simulink library "COR_lib"  (Simulink 7.4)
settings: Solver=FixedStepDiscrete  StartTime=0.0  StopTime=Inf  FixedStep=0.01  RelTol=1e-3
values from neighbouring files (symbols this model uses):
  CORc_fac_CellRDcse_fault = mpt.Parameter    [COR_CAL.m]
  CORc_fac_CellRDcse_warn = mpt.Parameter    [COR_CAL.m]
  CORc_i_ChaEndCur = mpt.Parameter    [COR_CAL.m]
  CORc_i_SOCCrectCurThrld = mpt.Parameter    [COR_CAL.m]
  CORc_pct_DeltSoe_max = mpt.Parameter    [COR_CAL.m]
  CORc_pct_DeltSoe_min = mpt.Parameter    [COR_CAL.m]
  CORc_pct_SOCModValue = mpt.Parameter    [COR_CAL.m]
  CORc_v_CellVoltMax = mpt.Parameter    [COR_CAL.m]
undefined symbols (not defined in the file or in its folder): BATd_iflt_CellCDcse_fault, BATd_pct_CellCVariMax, BATd_pct_CellCVariMin, BATd_v_CellUpperVolt, BATd_v_PackVoltMin, BATm_c_CellChaC_AH, BATm_c_CellDchC_AH, BATm_e_CellSoe, BATm_e_ChaCellSoe, BATm_e_DchCellSoe, BATm_i_PerChaCur, BATm_i_PerDchCur, BATm_i_PulChaCur_limit, BATm_i_PulDchCur_limit, BATm_i_PulDchVolt_limit, BATm_pct_CellCDcseRatio, BATm_pct_CellCycle, BATm_pct_CellSoc, BATm_pct_ChaCellSoc, BATm_pct_DchCellSoc, BATm_pct_SOCofOCVPct, BATm_pct_SohRatio, BATm_r_ChaDcIR, BATm_r_DchDcIR, BATm_v_CellOCV, BATx_pct_CellSocRatio, BATx_pct_PackSoh, BATx_t_CellChaTemp, BATx_t_CellDchTemp, BATx_tm_OfflineTime, BATy_i_CellChaCur, BATy_i_CellDchCur, BATz_v_CellChaVolt, BATz_v_DchCellVolt, BATz_v_DchCellVoltForSoe, BCU_FastCharge_St, BCU_SlowCharge_St, BMS_Const_TickTm_s, BMU_Run_St, FCM_Charging_St, PACK_Const_CellNumOfMdl, PACK_Const_CellNumOfPack, PACK_Const_CycCnt, PACK_Const_MdlNumOfPack, PACK_Const_ParaCellNumOfMdl, PACK_Const_TempSnrNumOfMdl, SCM_Charging_St
libraries: Defined_Functionality x17
(part 1 of 2)
settings Model: Creator=zhaoxiangri  LastModifiedBy=sunsijun

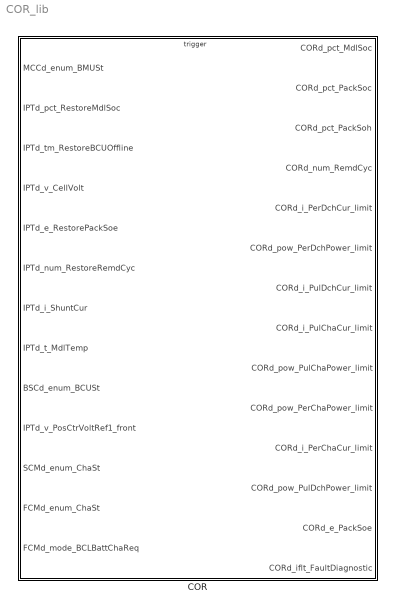
== system COR_lib ==
  COR : Subsystem  TreatAsAtomicUnit=on

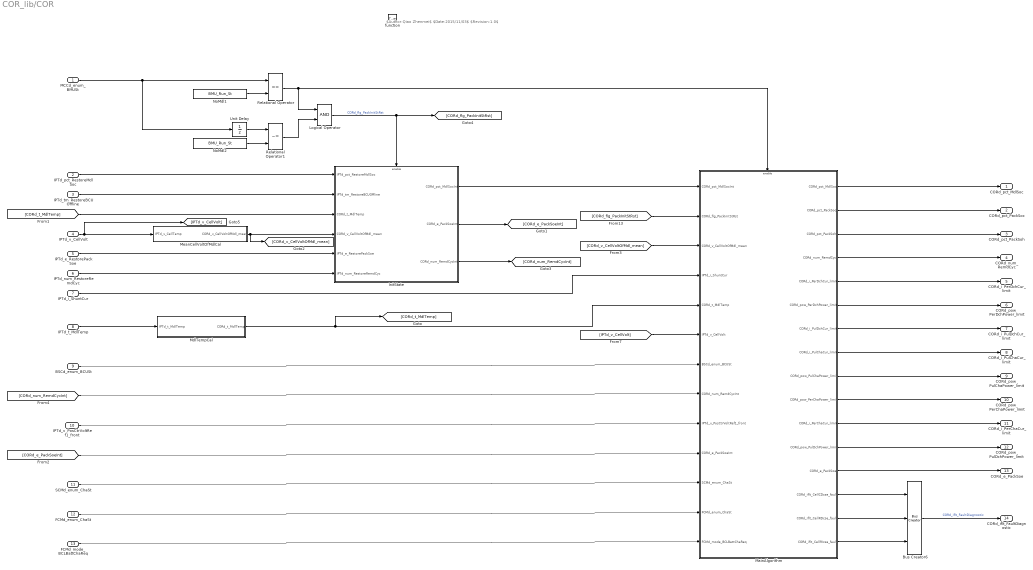
== system COR_lib/COR ==
  note: $Author:Qiao Zhenmei$
      | $Date:2015/11/03$
      | $Revision:1.0$
  MCCd_enum_BMUSt : Inport  OutDataType=sfix(16)  OutScaling=2^0
  IPTd_pct_RestoreMdlSoc : Inport  Port=2  OutDataType=sfix(16)  OutScaling=2^0
  IPTd_tm_RestoreBCUOffline : Inport  Port=3  OutDataType=sfix(16)  OutScaling=2^0
  IPTd_v_CellVolt : Inport  Port=4  OutDataType=sfix(16)  OutScaling=2^0
  IPTd_e_RestorePackSoe : Inport  Port=5  OutDataType=sfix(16)  OutScaling=2^0
  IPTd_num_RestoreRemdCyc : Inport  Port=6  OutDataType=sfix(16)  OutScaling=2^0
  IPTd_i_ShuntCur : Inport  Port=7
  IPTd_t_MdlTemp : Inport  Port=8  DataType=single  OutDataTypeStr=single
  BSCd_enum_BCUSt : Inport  Port=9
  IPTd_v_PosCtrVoltRef1_front : Inport  Port=10  OutDataType=fixdt(1,16,2^-6,0)
  SCMd_enum_ChaSt : Inport  Port=11
  FCMd_enum_ChaSt : Inport  Port=12
  FCMd_mode_BCLBattChaReq : Inport  Port=13
  function : TriggerPort  TriggerType=function-call
  Bus Creator6 : BusCreator  Inputs=3
  InitState : Subsystem
  Logical Operator : Logic  AllPortsSameDT=off  OutDataTypeMode=boolean  LogicDataType=fixdt(0, 8)  OutDataTypeStr=boolean
  MainAlgorithm : Subsystem
  MdlTempCal : Subsystem
  MeanCellVoltOfMdlCal : Subsystem
  NoMdl1 : Constant  Value=BMU_Run_St  OutDataTypeMode=uint8  OutDataType=fixdt(1, 16)  OutScaling=2^0  OutDataTypeStr=uint8
  NoMdl2 : Constant  Value=BMU_Run_St  OutDataTypeMode=uint8  OutDataType=fixdt(1, 16)  OutScaling=2^0  OutDataTypeStr=uint8
  Relational Operator : RelationalOperator  Operator===  LogicOutDataTypeMode=boolean  LogicDataType=fixdt(0, 8)  OutDataTypeStr=boolean
  Relational Operator1 : RelationalOperator  Operator=~=  LogicOutDataTypeMode=boolean  LogicDataType=fixdt(0, 8)  OutDataTypeStr=boolean
  Unit Delay : UnitDelay  SampleTime=-1
  CORd_pct_MdlSoc : Outport  InitialOutput=0
  CORd_pct_PackSoc : Outport  Port=2  InitialOutput=0
  CORd_pct_PackSoh : Outport  Port=3  InitialOutput=0
  CORd_num_RemdCyc : Outport  Port=4
  CORd_i_PerDchCur_limit : Outport  Port=5  InitialOutput=0
  CORd_pow_PerDchPower_limit : Outport  Port=6  InitialOutput=0
  CORd_i_PulDchCur_limit : Outport  Port=7  OutDataType=sfix(16)  OutScaling=2^0  InitialOutput=0
  CORd_i_PulChaCur_limit : Outport  Port=8  OutDataType=sfix(16)  OutScaling=2^0  InitialOutput=0
  CORd_pow_PulChaPower_limit : Outport  Port=9  OutDataType=sfix(16)  OutScaling=2^0  InitialOutput=0
  CORd_pow_PerChaPower_limit : Outport  Port=10  InitialOutput=0
  CORd_i_PerChaCur_limit : Outport  Port=11  InitialOutput=0
  CORd_pow_PulDchPower_limit : Outport  Port=12  OutDataType=sfix(16)  OutScaling=2^0  InitialOutput=0
  CORd_e_PackSoe : Outport  Port=13  InitialOutput=0
  CORd_iflt_FaultDiagnostic : Outport  Port=14
  wires:
  [CORd_num_RemdCycInt] -> MainAlgorithm/8(CORd_num_RemdCycInt)
  InitState/3(CORd_num_RemdCycInt) -> [CORd_num_RemdCycInt]
  [CORd_e_PackSoeInt] -> MainAlgorithm/10(CORd_e_PackSoeInt)
  InitState/2(CORd_e_PackSoeInt) -> [CORd_e_PackSoeInt]
  MainAlgorithm/16(CORd_iflt_CellRIcse_fault) -> Bus Creator6/3
  MainAlgorithm/15(CORd_iflt_CellRDcse_fault) -> Bus Creator6/2
  MainAlgorithm/14(CORd_iflt_CellCDcse_fault) -> Bus Creator6/1
  Relational Operator/1 -> Logical Operator/1, MainAlgorithm/Enable
  FCMd_enum_ChaSt/1 -> MainAlgorithm/12(FCMd_enum_ChaSt)
  SCMd_enum_ChaSt/1 -> MainAlgorithm/11(SCMd_enum_ChaSt)
  [IPTd_v_CellVolt] -> MainAlgorithm/6(IPTd_v_CellVolt)
  InitState/1(CORd_pct_MdlSocInt) -> MainAlgorithm/1(CORd_pct_MdlSocInt)
  IPTd_pct_RestoreMdlSoc/1 -> InitState/1(IPTd_pct_RestoreMdlSoc)
  IPTd_e_RestorePackSoe/1 -> InitState/5(IPTd_e_RestorePackSoe)
  IPTd_num_RestoreRemdCyc/1 -> InitState/6(IPTd_num_RestoreRemdCyc)
  [CORd_t_MdlTemp] -> InitState/3(CORd_t_MdlTemp)
  MCCd_enum_BMUSt/1 -> Unit Delay/1, Relational Operator/1
  Unit Delay/1 -> Relational Operator1/1
  NoMdl2/1 -> Relational Operator1/2
  Relational Operator1/1 -> Logical Operator/2
  Logical Operator/1 -> InitState/Enable, [CORd_flg_PackInitStRst]  "CORd_flg_PackInitStRst"
  IPTd_t_MdlTemp/1 -> MdlTempCal/1(IPTd_t_MdlTemp)
  MdlTempCal/1(CORd_t_MdlTemp) -> [CORd_t_MdlTemp], MainAlgorithm/5(CORd_t_MdlTemp)
  IPTd_v_PosCtrVoltRef1_front/1 -> MainAlgorithm/9(IPTd_v_PosCtrVoltRef1_front)
  MainAlgorithm/3(CORd_pct_PackSoh) -> CORd_pct_PackSoh/1
  MainAlgorithm/7(CORd_i_PulDchCur_limit) -> CORd_i_PulDchCur_limit/1
  MainAlgorithm/8(CORd_i_PulChaCur_limit) -> CORd_i_PulChaCur_limit/1
  MainAlgorithm/12(CORd_pow_PulDchPower_limit) -> CORd_pow_PulDchPower_limit/1
  MainAlgorithm/9(CORd_pow_PulChaPower_limit) -> CORd_pow_PulChaPower_limit/1
  MainAlgorithm/5(CORd_i_PerDchCur_limit) -> CORd_i_PerDchCur_limit/1
  MainAlgorithm/11(CORd_i_PerChaCur_limit) -> CORd_i_PerChaCur_limit/1
  MainAlgorithm/6(CORd_pow_PerDchPower_limit) -> CORd_pow_PerDchPower_limit/1
  MainAlgorithm/10(CORd_pow_PerChaPower_limit) -> CORd_pow_PerChaPower_limit/1
  [CORd_v_CellVoltOfMdl_mean] -> MainAlgorithm/3(CORd_v_CellVoltOfMdl_mean)
  IPTd_i_ShuntCur/1 -> MainAlgorithm/4(IPTd_i_ShuntCur)
  IPTd_tm_RestoreBCUOffline/1 -> InitState/2(IPTd_tm_RestoreBCUOffline)
  Bus Creator6/1 -> CORd_iflt_FaultDiagnostic/1  "CORd_iflt_FaultDiagnostic"
  NoMdl1/1 -> Relational Operator/2
  IPTd_v_CellVolt/1 -> [IPTd_v_CellVolt], MeanCellVoltOfMdlCal/1(IPTd_v_CellTemp)
  MeanCellVoltOfMdlCal/1(CORd_v_CellVoltOfMdl_mean) -> InitState/4(CORd_v_CellVoltOfMdl_mean), [CORd_v_CellVoltOfMdl_mean]
  FCMd_mode_BCLBattChaReq/1 -> MainAlgorithm/13(FCMd_mode_BCLBattChaReq)
  [CORd_flg_PackInitStRst] -> MainAlgorithm/2(CORd_flg_PackInitStRst)
  MainAlgorithm/1(CORd_pct_MdlSoc) -> CORd_pct_MdlSoc/1
  MainAlgorithm/2(CORd_pct_PackSoc) -> CORd_pct_PackSoc/1
  MainAlgorithm/13(CORd_e_PackSoe) -> CORd_e_PackSoe/1
  MainAlgorithm/4(CORd_num_RemdCyc) -> CORd_num_RemdCyc/1
  BSCd_enum_BCUSt/1 -> MainAlgorithm/7(BSCd_enum_BCUSt)

== system COR_lib/COR/InitState ==
  IPTd_pct_RestoreMdlSoc : Inport  OutDataType=sfix(16)  OutScaling=2^0
  IPTd_tm_RestoreBCUOffline : Inport  Port=2  OutDataType=sfix(16)  OutScaling=2^0
  CORd_t_MdlTemp : Inport  Port=3  OutDataType=sfix(16)  OutScaling=2^0
  CORd_v_CellVoltOfMdl_mean : Inport  Port=4  OutDataType=sfix(16)  OutScaling=2^0
  IPTd_e_RestorePackSoe : Inport  Port=5  OutDataType=sfix(16)  OutScaling=2^0
  IPTd_num_RestoreRemdCyc : Inport  Port=6  OutDataType=sfix(16)  OutScaling=2^0
  Enable : EnablePort
  SOCInit : Subsystem
  SOEInit : Subsystem
  SOHInit : Subsystem
  CORd_pct_MdlSocInt : Outport  OutDataType=fixdt(1, 16)  OutScaling=2^0
  CORd_e_PackSoeInt : Outport  Port=2  OutDataType=fixdt(1, 16)  OutScaling=2^0
  CORd_num_RemdCycInt : Outport  Port=3  OutDataType=fixdt(1, 16)  OutScaling=2^0
  wires:
  IPTd_e_RestorePackSoe/1 -> SOEInit/1(IPTd_v_RestorePackSoe)
  IPTd_pct_RestoreMdlSoc/1 -> SOCInit/1(IPTd_pct_RestoreMdlSoc)
  SOCInit/1(CORd_pct_MdlSocInt) -> CORd_pct_MdlSocInt/1
  IPTd_tm_RestoreBCUOffline/1 -> SOCInit/2(IPTd_tm_RestoreBCUOffline), [IPTd_tm_RestoreBCUOffline]
  CORd_v_CellVoltOfMdl_mean/1 -> SOCInit/4(CORd_v_CellVoltOfMdl_mean), [CORd_v_CellVoltOfMdl_mean]
  CORd_t_MdlTemp/1 -> SOCInit/3(CORd_t_MdlTemp), [CORd_t_MdlTemp]
  [IPTd_tm_RestoreBCUOffline] -> SOEInit/2(IPTd_tm_RestoreBCUOffline)
  [CORd_v_CellVoltOfMdl_mean] -> SOEInit/3(CORd_v_CellVoltOfMdl_mean)
  [CORd_t_MdlTemp] -> SOEInit/4(CORd_t_MdlTemp)
  SOEInit/1(CORd_e_PackSoeInt) -> CORd_e_PackSoeInt/1
  SOHInit/1(CORd_num_RemdCycInt) -> CORd_num_RemdCycInt/1
  IPTd_num_RestoreRemdCyc/1 -> SOHInit/1(IPTd_num_RestoreRemdCyc)

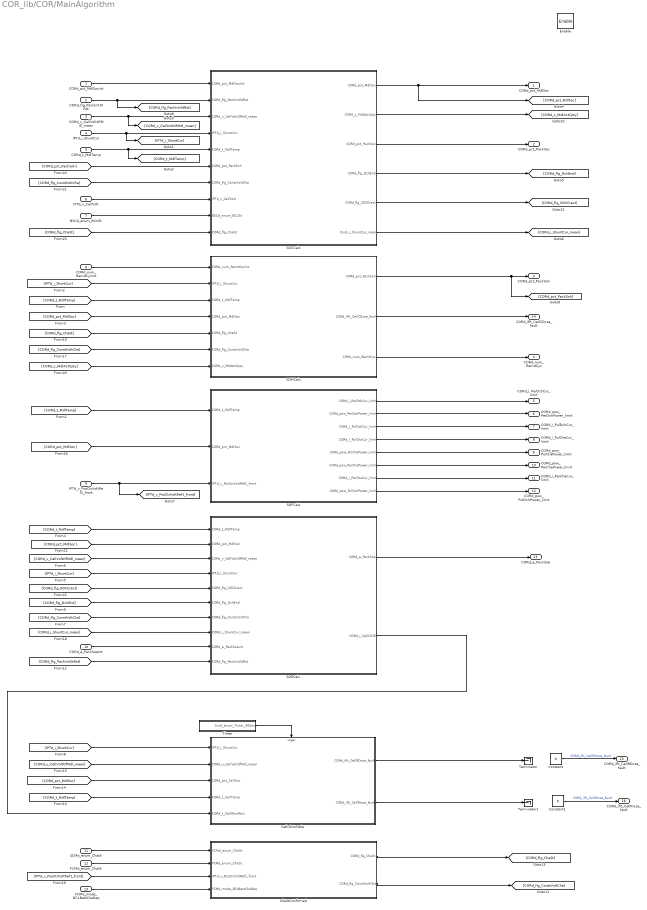
== system COR_lib/COR/MainAlgorithm ==
  CORd_pct_MdlSocInt : Inport
  CORd_flg_PackInitStRst : Inport  Port=2
  CORd_v_CellVoltOfMdl_mean : Inport  Port=3
  IPTd_i_ShuntCur : Inport  Port=4
  CORd_t_MdlTemp : Inport  Port=5
  IPTd_v_CellVolt : Inport  Port=6
  BSCd_enum_BCUSt : Inport  Port=7
  CORd_num_RemdCycInt : Inport  Port=8
  IPTd_v_PosCtrVoltRef1_front : Inport  Port=9
  CORd_e_PackSoeInt : Inport  Port=10
  SCMd_enum_ChaSt : Inport  Port=11
  FCMd_enum_ChaSt : Inport  Port=12
  FCMd_mode_BCLBattChaReq : Inport  Port=13
  Enable : EnablePort
  CellOhmRObs : Subsystem
  ChaStConfirmed : Subsystem
  Constant : Constant  Value=0  OutDataTypeMode=boolean  OutDataType=fixdt(1, 16)  OutScaling=2^0  OutDataTypeStr=boolean
  Constant1 : Constant  Value=0  OutDataTypeMode=boolean  OutDataType=fixdt(1, 16)  OutScaling=2^0  OutDataTypeStr=boolean
  SOCCalc : Subsystem
  SOECalc : Subsystem
  SOFCalc : Subsystem
  SOHCalc : Subsystem  TreatAsAtomicUnit=on
  Terminator : Terminator
  Terminator1 : Terminator
  Timer : Subsystem
  CORd_pct_MdlSoc : Outport
  CORd_pct_PackSoc : Outport  Port=2
  CORd_pct_PackSoh : Outport  Port=3
  CORd_num_RemdCyc : Outport  Port=4  OutDataType=fixdt(1, 16)  OutScaling=2^0  InitialOutput=0
  CORd_i_PerDchCur_limit : Outport  Port=5
  CORd_pow_PerDchPower_limit : Outport  Port=6
  CORd_i_PulDchCur_limit : Outport  Port=7  OutDataType=sfix(16)  OutScaling=2^0
  CORd_i_PulChaCur_limit : Outport  Port=8  OutDataType=sfix(16)  OutScaling=2^0
  CORd_pow_PulChaPower_limit : Outport  Port=9  OutDataType=sfix(16)  OutScaling=2^0
  CORd_pow_PerChaPower_limit : Outport  Port=10
  CORd_i_PerChaCur_limit : Outport  Port=11
  CORd_pow_PulDchPower_limit : Outport  Port=12  OutDataType=sfix(16)  OutScaling=2^0
  CORd_e_PackSoe : Outport  Port=13
  CORd_iflt_CellCDcse_fault : Outport  Port=14  OutDataType=fixdt(1, 16)  OutScaling=2^0  InitialOutput=0
  CORd_iflt_CellRDcse_fault : Outport  Port=15  OutDataType=fixdt(1, 16)  OutScaling=2^0  InitialOutput=0
  CORd_iflt_CellRIcse_fault : Outport  Port=16  OutDataType=fixdt(1, 16)  OutScaling=2^0  InitialOutput=0
  wires:
  [CORd_pct_PackSoh] -> SOCCalc/6(CORd_pct_PackSoh)
  CORd_v_CellVoltOfMdl_mean/1 -> [CORd_v_CellVoltOfMdl_mean], SOCCalc/3(CORd_v_CellVoltOfMdl_mean)
  SOCCalc/1(CORd_pct_MdlSoc) -> [CORd_pct_MdlSoc], CORd_pct_MdlSoc/1
  ChaStConfirmed/1(CORd_flg_ChaSt) -> [CORd_flg_ChaSt]
  IPTd_i_ShuntCur/1 -> [IPTd_i_ShuntCur], SOCCalc/4(IPTd_i_ShuntCur)
  [CORd_flg_ChaSt] -> SOHCalc/5(CORd_flg_ChaSt)
  [CORd_flg_ChaSt] -> SOCCalc/10(CORd_flg_ChaSt)
  FCMd_enum_ChaSt/1 -> ChaStConfirmed/2(FCMd_enum_ChaSt)
  SCMd_enum_ChaSt/1 -> ChaStConfirmed/1(SCMd_enum_ChaSt)
  [CORd_flg_SOCCrect] -> SOECalc/5(CORd_flg_SOCCrect)
  SOCCalc/5(CORd_flg_SOCCrect) -> [CORd_flg_SOCCrect]
  [CORd_flg_ConstVoltCha] -> SOCCalc/7(CORd_flg_ConstVoltCha)
  IPTd_v_CellVolt/1 -> SOCCalc/8(IPTd_v_CellVolt)
  [CORd_c_MdlActCpty] -> SOHCalc/7(CORd_c_MdlActCpty)
  SOCCalc/2(CORd_c_MdlActCpty) -> [CORd_c_MdlActCpty]
  [CORd_i_ShuntCur_mean] -> SOECalc/8(CORd_i_ShuntCur_mean)
  SOCCalc/6(Cord_i_ShuntCur_mean) -> [CORd_i_ShuntCur_mean]
  [CORd_t_MdlTemp] -> SOHCalc/3(CORd_t_MdlTemp)
  [CORd_t_MdlTemp] -> SOFCalc/1(CORd_t_MdlTemp)
  SOFCalc/3(CORd_i_PulDchCur_limit) -> CORd_i_PulDchCur_limit/1
  SOFCalc/4(CORd_i_PulChaCur_limit) -> CORd_i_PulChaCur_limit/1
  SOFCalc/8(CORd_pow_PulDchPower_limit) -> CORd_pow_PulDchPower_limit/1
  SOFCalc/5(CORd_pow_PulChaPower_limit) -> CORd_pow_PulChaPower_limit/1
  CORd_t_MdlTemp/1 -> [CORd_t_MdlTemp], SOCCalc/5(CORd_t_MdlTemp)
  [IPTd_i_ShuntCur] -> SOECalc/4(IPTd_i_ShuntCur)
  [CORd_t_MdlTemp] -> SOECalc/1(CORd_t_MdlTemp)
  [CORd_v_CellVoltOfMdl_mean] -> SOECalc/3(CORd_v_CellVoltOfMdl_mean)
  [CORd_pct_MdlSoc] -> SOHCalc/4(CORd_pct_MdlSoc)
  IPTd_v_PosCtrVoltRef1_front/1 -> SOFCalc/3(IPTd_v_PosCtrVoltRef1_front), [IPTd_v_PosCtrVoltRef1_front]
  SOFCalc/1(CORd_i_PerDchCur_limit) -> CORd_i_PerDchCur_limit/1
  SOFCalc/7(CORd_i_PerChaCur_limit) -> CORd_i_PerChaCur_limit/1
  SOFCalc/2(CORd_pow_PerDchPower_limit) -> CORd_pow_PerDchPower_limit/1
  SOFCalc/6(CORd_pow_PerChaPower_limit) -> CORd_pow_PerChaPower_limit/1
  SOCCalc/4(CORd_flg_DchEnd) -> [CORd_flg_DchEnd]
  [CORd_flg_DchEnd] -> SOECalc/6(CORd_flg_DchEnd)
  [CORd_pct_MdlSoc] -> SOECalc/2(CORd_pct_MdlSoc)
  [CORd_flg_ConstVoltCha] -> SOECalc/7(CORd_flg_ConstVoltCha)
  SOECalc/1(CORd_e_PackSoe) -> CORd_e_PackSoe/1
  [CORd_flg_ConstVoltCha] -> SOHCalc/6(CORd_flg_ConstVoltCha)
  SOHCalc/2(CORd_iflt_CellCDcse_fault) -> CORd_iflt_CellCDcse_fault/1
  [IPTd_i_ShuntCur] -> CellOhmRObs/1(IPTd_i_ShuntCur)
  [CORd_v_CellVoltOfMdl_mean] -> CellOhmRObs/2(CORd_v_CellVoltOfMdl_mean)
  [CORd_pct_MdlSoc] -> CellOhmRObs/3(CORd_pct_CellSoc)
  [CORd_t_MdlTemp] -> CellOhmRObs/4(CORd_t_CellTemp)
  Constant/1 -> CORd_iflt_CellRDcse_fault/1  "CORd_iflt_CellRDcse_fault"
  Constant1/1 -> CORd_iflt_CellRIcse_fault/1  "CORd_iflt_CellRIcse_fault"
  CellOhmRObs/1(CORd_iflt_CellRDcse_fault) -> Terminator/1
  CellOhmRObs/2(CORd_iflt_CellRIcse_fault) -> Terminator1/1
  SOECalc/2(CORd_r_CellDCIR) -> CellOhmRObs/5(CORd_t_CellOhmRInt)
  [CORd_pct_MdlSoc] -> SOFCalc/2(CORd_pct_MdlSoc)
  SOHCalc/1(CORd_pct_PackSoh) -> [CORd_pct_PackSoh], CORd_pct_PackSoh/1
  Timer/1(Cord_enum_Timer_300ms) -> CellOhmRObs/Trigger
  ChaStConfirmed/2(CORd_flg_ConstVoltCha) -> [CORd_flg_ConstVoltCha]
  [IPTd_v_PosCtrVoltRef1_front] -> ChaStConfirmed/3(IPTd_v_PosCtrVoltRef1_front)
  FCMd_mode_BCLBattChaReq/1 -> ChaStConfirmed/4(FCMd_mode_BCLBattChaReq)
  SOCCalc/3(CORd_pct_PackSoc) -> CORd_pct_PackSoc/1
  CORd_pct_MdlSocInt/1 -> SOCCalc/1(CORd_pct_MdlSocInt)
  CORd_flg_PackInitStRst/1 -> SOCCalc/2(CORd_flg_PackInitStRst), [CORd_flg_PackInitStRst]
  CORd_e_PackSoeInt/1 -> SOECalc/9(CORd_e_PackSoeInt)
  [CORd_flg_PackInitStRst] -> SOECalc/10(CORd_flg_PackInitStRst)
  [IPTd_i_ShuntCur] -> SOHCalc/2(IPTd_i_ShuntCur)
  CORd_num_RemdCycInt/1 -> SOHCalc/1(CORd_num_RemdCycInt)
  SOHCalc/3(CORd_num_RemdCyc) -> CORd_num_RemdCyc/1
  BSCd_enum_BCUSt/1 -> SOCCalc/9(BSCd_enum_BCUSt)

== system COR_lib/COR/MdlTempCal ==
  IPTd_t_MdlTemp : Inport
  Constant : Constant  Value=PACK_Const_TempSnrNumOfMdl  OutDataTypeMode=single  OutDataType=fixdt(1, 16)  OutScaling=2^0  OutDataTypeStr=single
  Divide : Product  Inputs=*/  OutDataType=fixdt(1,16,2^-5,0)
  Reshape : Reshape  OutputDimensionality=Customize  OutputDimensions=[2,32]
  Sum of Elements : Sum  Inputs=+  CollapseMode=Specified dimension  OutDataType=fixdt(1,16,2^-7,150)
  saturation : Defined_Functionality/saturation  SystemSampleTime=-1  upper_limit=60  lower_limit=-40
      settings: AttributesFormatString=[UPPER_LIMIT=%<upper_limit>]\n[LOWER_LIMIT=%<lower_limit>]
  CORd_t_MdlTemp : Outport
  wires:
  Sum of Elements/1 -> Divide/1
  Constant/1 -> Divide/2
  IPTd_t_MdlTemp/1 -> Reshape/1
  Divide/1 -> saturation/1
  Reshape/1 -> Sum of Elements/1
  saturation/1 -> CORd_t_MdlTemp/1  "CORd_t_MdlTemp"

== system COR_lib/COR/MeanCellVoltOfMdlCal ==
  IPTd_v_CellTemp : Inport
  Constant1 : Constant  Value=PACK_Const_CellNumOfMdl  OutDataTypeMode=uint8  OutDataType=fixdt(1, 16)  OutScaling=2^0  OutDataTypeStr=uint8
  Divide : Product  Inputs=*/  OutDataType=fixdt(1, 16)  OutScaling=2^-10
  Reshape : Reshape  OutputDimensionality=Customize  OutputDimensions=[5,32]
  Sum of Elements : Sum  Inputs=+  CollapseMode=Specified dimension  OutDataType=fixdt(1, 16)  OutScaling=2^-10  OutDataTypeStr=Inherit: Inherit via back propagation
  CORd_v_CellVoltOfMdl_mean : Outport
  wires:
  Sum of Elements/1 -> Divide/1
  Constant1/1 -> Divide/2
  IPTd_v_CellTemp/1 -> Reshape/1
  Divide/1 -> CORd_v_CellVoltOfMdl_mean/1  "CORd_v_CellVoltOfMdl_mean"
  Reshape/1 -> Sum of Elements/1

== system COR_lib/COR/InitState/SOCInit ==
  IPTd_pct_RestoreMdlSoc : Inport  OutDataType=sfix(16)  OutScaling=2^0
  IPTd_tm_RestoreBCUOffline : Inport  Port=2  DataType=single  OutDataType=sfix(16)  OutScaling=2^0  OutDataTypeStr=single
  CORd_t_MdlTemp : Inport  Port=3  OutDataType=sfix(16)  OutScaling=2^0
  CORd_v_CellVoltOfMdl_mean : Inport  Port=4  OutDataType=sfix(16)  OutScaling=2^0
  Add : Sum  OutDataType=fixdt(1, 16)  OutScaling=2^-10
  COR_SocInt : Lookup  InputValues=BATx_tm_OfflineTime  Table=BATm_pct_SOCofOCVPct  LookUpMeth=Interpolation-Use End Values  OutDataTypeMode=single  OutDataType=sfix(16)  OutScaling=2^0  OutDataTypeStr=single
  Constant : Constant  OutDataTypeMode=single  OutDataType=fixdt(1, 16)  OutScaling=2^0  OutDataTypeStr=single
  Product : Product  OutDataType=fixdt(1, 16)  OutScaling=2^0  RndMeth=Zero
  Product1 : Product  OutDataType=fixdt(1, 16)  OutScaling=2^0  RndMeth=Zero
  Subtract : Sum  Inputs=+-  OutDataType=fixdt(1, 16)  OutScaling=2^-10
  T-OCV-SOC_Curve : Lookup2D  RowIndex=BATx_t_CellTemp  ColumnIndex=BATy_v_CellOCV  Table=BATm_pct_CellSoc  LookUpMeth=Interpolation-Use End Values  OutDataType=fixdt(1, 16)  OutScaling=2^0
  saturation : Defined_Functionality/saturation  SystemSampleTime=-1  upper_limit=1  lower_limit=0
      settings: AttributesFormatString=[UPPER_LIMIT=%<upper_limit>]\n[LOWER_LIMIT=%<lower_limit>]
  CORd_pct_MdlSocInt : Outport  OutDataType=fixdt(1, 16)  OutScaling=2^0
  wires:
  saturation/1 -> Product/1, Subtract/2
  IPTd_tm_RestoreBCUOffline/1 -> COR_SocInt/1
  CORd_t_MdlTemp/1 -> T-OCV-SOC_Curve/1
  CORd_v_CellVoltOfMdl_mean/1 -> T-OCV-SOC_Curve/2
  COR_SocInt/1 -> saturation/1
  T-OCV-SOC_Curve/1 -> Product/2
  Constant/1 -> Subtract/1
  IPTd_pct_RestoreMdlSoc/1 -> Product1/1
  Subtract/1 -> Product1/2
  Product1/1 -> Add/1
  Product/1 -> Add/2
  Add/1 -> CORd_pct_MdlSocInt/1  "CORd_pct_MdlSocInt"

== system COR_lib/COR/InitState/SOEInit ==
  IPTd_v_RestorePackSoe : Inport  OutDataType=sfix(16)  OutScaling=2^0
  IPTd_tm_RestoreBCUOffline : Inport  Port=2  OutDataType=sfix(16)  OutScaling=2^0
  CORd_v_CellVoltOfMdl_mean : Inport  Port=3  OutDataType=sfix(16)  OutScaling=2^0
  CORd_t_MdlTemp : Inport  Port=4  OutDataType=sfix(16)  OutScaling=2^0
  Add : Sum  OutDataType=fixdt(1, 16)  OutScaling=2^-10
  COR_SoeInit : Lookup  InputValues=BATx_tm_OfflineTime  Table=BATm_pct_SOCofOCVPct  LookUpMeth=Interpolation-Use End Values  OutDataTypeMode=single  OutDataType=sfix(16)  OutScaling=2^0  OutDataTypeStr=single
  Constant : Constant  OutDataTypeMode=single  OutDataType=fixdt(1, 16)  OutScaling=2^0  OutDataTypeStr=single
  Constant1 : Constant  Value=PACK_Const_ParaCellNumOfMdl  OutDataTypeMode=uint8  OutDataType=fixdt(1, 16)  OutScaling=2^0  OutDataTypeStr=uint8
  Constant2 : Constant  Value=PACK_Const_CellNumOfMdl  OutDataTypeMode=uint8  OutDataType=fixdt(1, 16)  OutScaling=2^0  OutDataTypeStr=uint8
  Gain : Gain  Gain=1000  ParameterDataType=fixdt(1, 16)  ParameterScaling=2^0  OutDataType=fixdt(1, 16)  OutScaling=2^0
  Product{,1..3} (4 alike) : Product  OutDataType=fixdt(1, 16)  OutScaling=2^0  RndMeth=Zero
  Subtract : Sum  Inputs=+-  OutDataType=fixdt(1, 16)  OutScaling=2^-10
  Sum of Elements : Sum  Inputs=+  OutDataType=fixdt(1, 16)  OutScaling=2^-10
  T-OCV-SOE_Curve : Lookup2D  RowIndex=BATx_t_CellTemp  ColumnIndex=BATy_v_CellOCV  Table=BATm_e_CellSoe  LookUpMeth=Interpolation-Use End Values  OutDataType=fixdt(1, 16)  OutScaling=2^0
  saturation : Defined_Functionality/saturation  SystemSampleTime=-1  upper_limit=1  lower_limit=0
      settings: AttributesFormatString=[UPPER_LIMIT=%<upper_limit>]\n[LOWER_LIMIT=%<lower_limit>]
  CORd_e_PackSoeInt : Outport  OutDataType=fixdt(1, 16)  OutScaling=2^0
  wires:
  saturation/1 -> Product/1, Subtract/2
  IPTd_tm_RestoreBCUOffline/1 -> COR_SoeInit/1
  CORd_t_MdlTemp/1 -> T-OCV-SOE_Curve/1
  CORd_v_CellVoltOfMdl_mean/1 -> T-OCV-SOE_Curve/2
  COR_SoeInit/1 -> saturation/1
  T-OCV-SOE_Curve/1 -> Product/2
  Constant/1 -> Subtract/1
  IPTd_v_RestorePackSoe/1 -> Gain/1
  Subtract/1 -> Product1/2
  Product1/1 -> Add/1
  Add/1 -> CORd_e_PackSoeInt/1  "CORd_e_PackSoeInt"
  Gain/1 -> Product1/1
  Sum of Elements/1 -> Add/2
  Product/1 -> Product2/1
  Product2/1 -> Sum of Elements/1
  Constant1/1 -> Product3/1
  Constant2/1 -> Product3/2
  Product3/1 -> Product2/2

== system COR_lib/COR/InitState/SOHInit ==
  IPTd_num_RestoreRemdCyc : Inport
  Gain : Gain  ParameterDataType=fixdt(1, 16)  ParameterScaling=2^0  OutDataType=fixdt(1, 16)  OutScaling=2^0
  CORd_num_RemdCycInt : Outport
  wires:
  IPTd_num_RestoreRemdCyc/1 -> Gain/1
  Gain/1 -> CORd_num_RemdCycInt/1  "CORd_num_RemdCycInt"

== system COR_lib/COR/MainAlgorithm/CellOhmRObs ==
  IPTd_i_ShuntCur : Inport
  CORd_v_CellVoltOfMdl_mean : Inport  Port=2
  CORd_pct_CellSoc : Inport  Port=3
  CORd_t_CellTemp : Inport  Port=4
  CORd_t_CellOhmRInt : Inport  Port=5
  Trigger : TriggerPort
  CellOhmRCal : Subsystem
  CellOhmRObs : Subsystem
  Timer : Subsystem
  CORd_iflt_CellRDcse_fault : Outport  OutDataType=fixdt(1, 16)  OutScaling=2^0
  CORd_iflt_CellRIcse_fault : Outport  Port=2  OutDataType=fixdt(1, 16)  OutScaling=2^0
  wires:
  CellOhmRObs/1(CORd_iflt_CellRDcse_fault) -> CORd_iflt_CellRDcse_fault/1
  CellOhmRObs/2(CORd_iflt_CellRIcse_fault) -> CORd_iflt_CellRIcse_fault/1
  CORd_v_CellVoltOfMdl_mean/1 -> CellOhmRCal/2(CORd_v_CellVoltOfMdl_mean)
  CORd_pct_CellSoc/1 -> CellOhmRCal/3(CORd_pct_CellSoc)
  CORd_t_CellTemp/1 -> CellOhmRCal/4(CORd_t_CellTemp)
  IPTd_i_ShuntCur/1 -> CellOhmRCal/1(IPTd_i_ShuntCur)
  CellOhmRCal/1(CORd_r_CellOhmR) -> CellOhmRObs/1(CORd_r_CellOhmR)
  CORd_t_CellOhmRInt/1 -> CellOhmRObs/2(CORd_r_CellOhmRInt)
  Timer/1(Cord_flag_CellOhmRObs) -> CellOhmRObs/Enable

== system COR_lib/COR/MainAlgorithm/ChaStConfirmed ==
  SCMd_enum_ChaSt : Inport
  FCMd_enum_ChaSt : Inport  Port=2
  IPTd_v_PosCtrVoltRef1_front : Inport  Port=3
  FCMd_mode_BCLBattChaReq : Inport  Port=4
  Constant1 : Constant  Value=663  OutDataTypeMode=single  OutDataType=fixdt(1, 16)  OutScaling=2^0  OutDataTypeStr=single
  Constant2 : Constant  Value=SCM_Charging_St  OutDataType=fixdt(1, 16)  OutScaling=2^0
  Constant3 : Constant  Value=FCM_Charging_St  OutDataType=fixdt(1, 16)  OutScaling=2^0
  Constant4 : Constant  OutDataTypeMode=single  OutDataType=fixdt(1, 16)  OutScaling=2^0  OutDataTypeStr=single
  Logical Operator1 : Logic  Operator=OR  AllPortsSameDT=off  OutDataTypeMode=boolean  LogicDataType=fixdt(0, 8)  OutDataTypeStr=boolean
  Logical Operator2 : Logic  AllPortsSameDT=off  OutDataTypeMode=boolean  LogicDataType=fixdt(0, 8)  OutDataTypeStr=boolean
  Logical Operator3 : Logic  Operator=OR  AllPortsSameDT=off  OutDataTypeMode=boolean  LogicDataType=fixdt(0, 8)  OutDataTypeStr=boolean
  Logical Operator5 : Logic  AllPortsSameDT=off  OutDataTypeMode=boolean  LogicDataType=fixdt(0, 8)  OutDataTypeStr=boolean
  Relational Operator : RelationalOperator  LogicOutDataTypeMode=boolean  LogicDataType=fixdt(0, 8)  OutDataTypeStr=boolean
  Relational Operator1 : RelationalOperator  Operator===  LogicOutDataTypeMode=boolean  LogicDataType=fixdt(0, 8)  OutDataTypeStr=boolean
  Relational Operator2 : RelationalOperator  Operator===  LogicOutDataTypeMode=boolean  LogicDataType=fixdt(0, 8)  OutDataTypeStr=boolean
  Relational Operator3 : RelationalOperator  Operator===  LogicOutDataTypeMode=boolean  LogicDataType=fixdt(0, 8)  OutDataTypeStr=boolean
  CORd_flg_ChaSt : Outport
  CORd_flg_ConstVoltCha : Outport  Port=2
  wires:
  [CORd_flg_ChaSt] -> Logical Operator2/1
  Logical Operator3/1 -> [CORd_flg_ChaSt], Logical Operator5/1, CORd_flg_ChaSt/1  "CORd_flg_ChaSt"
  Relational Operator3/1 -> Logical Operator3/2
  Relational Operator2/1 -> Logical Operator3/1
  Constant2/1 -> Relational Operator2/2
  Constant3/1 -> Relational Operator3/2
  FCMd_enum_ChaSt/1 -> Relational Operator3/1
  SCMd_enum_ChaSt/1 -> Relational Operator2/1
  Logical Operator2/1 -> Logical Operator1/2
  Relational Operator1/1 -> Logical Operator2/2
  Logical Operator5/1 -> Logical Operator1/1
  Constant1/1 -> Relational Operator/2
  IPTd_v_PosCtrVoltRef1_front/1 -> Relational Operator/1
  Logical Operator1/1 -> CORd_flg_ConstVoltCha/1  "CORd_flg_ConstVoltCha"
  FCMd_mode_BCLBattChaReq/1 -> Relational Operator1/1
  Constant4/1 -> Relational Operator1/2
  Relational Operator/1 -> Logical Operator5/2

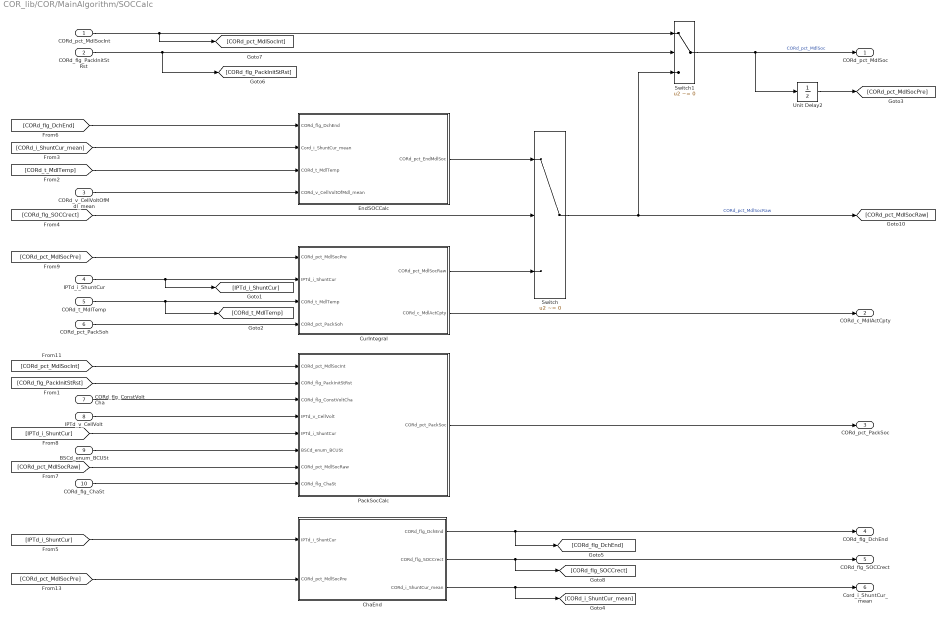
== system COR_lib/COR/MainAlgorithm/SOCCalc ==
  CORd_pct_MdlSocInt : Inport
  CORd_flg_PackInitStRst : Inport  Port=2
  CORd_v_CellVoltOfMdl_mean : Inport  Port=3
  IPTd_i_ShuntCur : Inport  Port=4
  CORd_t_MdlTemp : Inport  Port=5
  CORd_pct_PackSoh : Inport  Port=6
  CORd_flg_ConstVoltCha : Inport  Port=7
  IPTd_v_CellVolt : Inport  Port=8
  BSCd_enum_BCUSt : Inport  Port=9
  CORd_flg_ChaSt : Inport  Port=10
  ChaEnd : Subsystem
  CurIntegral : Subsystem
  EndSOCCalc : Subsystem
  PackSocCalc : Subsystem
  Switch : Switch  Criteria=u2 ~= 0  OutDataType=fixdt(1, 16)  OutScaling=2^0  OutDataTypeStr=Inherit: Inherit via back propagation
  Switch1 : Switch  Criteria=u2 ~= 0  OutDataType=fixdt(1, 16)  OutScaling=2^0
  Unit Delay2 : UnitDelay  SampleTime=-1
  CORd_pct_MdlSoc : Outport
  CORd_c_MdlActCpty : Outport  Port=2
  CORd_pct_PackSoc : Outport  Port=3
  CORd_flg_DchEnd : Outport  Port=4
  CORd_flg_SOCCrect : Outport  Port=5
  Cord_i_ShuntCur_mean : Outport  Port=6
  wires:
  [CORd_flg_PackInitStRst] -> PackSocCalc/2(CORd_flg_PackInitStRst)
  [CORd_pct_MdlSocInt] -> PackSocCalc/1(CORd_pct_MdlSocInt)
  PackSocCalc/1(CORd_pct_PackSoc) -> CORd_pct_PackSoc/1
  [CORd_pct_MdlSocRaw] -> PackSocCalc/7(CORd_pct_MdlSocRaw)
  EndSOCCalc/1(CORd_pct_EndMdlSoc) -> Switch/1
  CORd_flg_PackInitStRst/1 -> [CORd_flg_PackInitStRst], Switch1/2
  ChaEnd/3(CORd_i_ShuntCur_mean) -> [CORd_i_ShuntCur_mean], Cord_i_ShuntCur_mean/1
  ChaEnd/2(CORd_flg_SOCCrect) -> [CORd_flg_SOCCrect], CORd_flg_SOCCrect/1
  CORd_flg_ChaSt/1 -> PackSocCalc/8(CORd_flg_ChaSt)
  CORd_flg_ConstVoltCha/1 -> PackSocCalc/3(CORd_flg_ConstVoltCha)
  IPTd_v_CellVolt/1 -> PackSocCalc/4(IPTd_v_CellVolt)
  Switch/1 -> [CORd_pct_MdlSocRaw], Switch1/3  "CORd_pct_MdlSocRaw"
  [CORd_flg_SOCCrect] -> Switch/2
  CurIntegral/1(CORd_pct_MdlSocRaw) -> Switch/3
  [IPTd_i_ShuntCur] -> PackSocCalc/5(IPTd_i_ShuntCur)
  Unit Delay2/1 -> [CORd_pct_MdlSocPre]
  Switch1/1 -> Unit Delay2/1, CORd_pct_MdlSoc/1  "CORd_pct_MdlSoc"
  CORd_pct_MdlSocInt/1 -> [CORd_pct_MdlSocInt], Switch1/1
  BSCd_enum_BCUSt/1 -> PackSocCalc/6(BSCd_enum_BCUSt)
  [CORd_i_ShuntCur_mean] -> EndSOCCalc/2(Cord_i_ShuntCur_mean)
  CurIntegral/2(CORd_c_MdlActCpty) -> CORd_c_MdlActCpty/1
  IPTd_i_ShuntCur/1 -> [IPTd_i_ShuntCur], CurIntegral/2(IPTd_i_ShuntCur)
  CORd_t_MdlTemp/1 -> [CORd_t_MdlTemp], CurIntegral/3(CORd_t_MdlTemp)
  [CORd_t_MdlTemp] -> EndSOCCalc/3(CORd_t_MdlTemp)
  CORd_v_CellVoltOfMdl_mean/1 -> EndSOCCalc/4(CORd_v_CellVoltOfMdl_mean)
  CORd_pct_PackSoh/1 -> CurIntegral/4(CORd_pct_PackSoh)
  [IPTd_i_ShuntCur] -> ChaEnd/1(IPTd_i_ShuntCur)
  [CORd_pct_MdlSocPre] -> ChaEnd/2(CORd_pct_MdlSocPre)
  [CORd_flg_DchEnd] -> EndSOCCalc/1(CORd_flg_DchEnd)
  ChaEnd/1(CORd_flg_DchEnd) -> [CORd_flg_DchEnd], CORd_flg_DchEnd/1
  [CORd_pct_MdlSocPre] -> CurIntegral/1(CORd_pct_MdlSocPre)

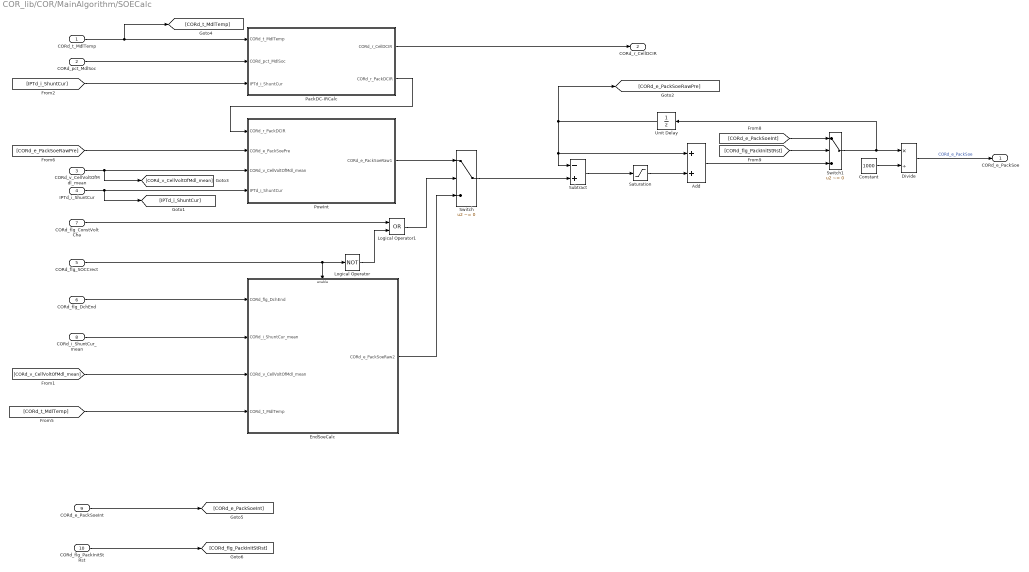
== system COR_lib/COR/MainAlgorithm/SOECalc ==
  CORd_t_MdlTemp : Inport
  CORd_pct_MdlSoc : Inport  Port=2
  CORd_v_CellVoltOfMdl_mean : Inport  Port=3
  IPTd_i_ShuntCur : Inport  Port=4
  CORd_flg_SOCCrect : Inport  Port=5
  CORd_flg_DchEnd : Inport  Port=6
  CORd_flg_ConstVoltCha : Inport  Port=7
  CORd_i_ShuntCur_mean : Inport  Port=8
  CORd_e_PackSoeInt : Inport  Port=9
  CORd_flg_PackInitStRst : Inport  Port=10
  Add : Sum  OutDataTypeMode=single  OutDataType=fixdt(1, 16)  OutScaling=2^-10  OutDataTypeStr=single
  Constant : Constant  Value=1000  OutDataTypeMode=uint16  OutDataType=fixdt(1, 16)  OutScaling=2^0  OutDataTypeStr=uint16
  Divide : Product  Inputs=*/  OutDataType=fixdt(1, 16)  OutScaling=2^-10
  EndSoeCalc : Subsystem
  Logical Operator : Logic  Operator=NOT  AllPortsSameDT=off  OutDataTypeMode=boolean  LogicDataType=fixdt(0, 8)  OutDataTypeStr=boolean
  Logical Operator1 : Logic  Operator=OR  AllPortsSameDT=off  OutDataTypeMode=boolean  LogicDataType=fixdt(0, 8)  OutDataTypeStr=boolean
  PackDC-IRCalc : Subsystem
  PowInt : Subsystem
  Saturation : Saturate  UpperLimit=CORc_pct_DeltSoe_max  LowerLimit=CORc_pct_DeltSoe_min  OutDataTypeMode=single  OutDataType=fixdt(1, 16)  OutScaling=2^0  OutDataTypeStr=single
  Subtract : Sum  Inputs=-+  OutDataTypeMode=single  OutDataType=fixdt(1, 16)  OutScaling=2^-10  OutDataTypeStr=single
  Switch : Switch  Criteria=u2 ~= 0  OutDataType=fixdt(1, 16)  OutScaling=2^0
  Switch1 : Switch  Criteria=u2 ~= 0  OutDataType=fixdt(1, 16)  OutScaling=2^0
  Unit Delay : UnitDelay  SampleTime=-1
  CORd_e_PackSoe : Outport
  CORd_r_CellDCIR : Outport  Port=2
  wires:
  Logical Operator1/1 -> Switch/2
  Logical Operator/1 -> Logical Operator1/2
  CORd_flg_ConstVoltCha/1 -> Logical Operator1/1
  Add/1 -> Switch1/3
  CORd_i_ShuntCur_mean/1 -> EndSoeCalc/2(CORd_i_ShuntCur_mean)
  EndSoeCalc/1(CORd_e_PackSoeRaw2) -> Switch/3
  CORd_flg_SOCCrect/1 -> EndSoeCalc/Enable, Logical Operator/1
  [CORd_e_PackSoeRawPre] -> PowInt/2(CORd_e_PackSoePre)
  CORd_v_CellVoltOfMdl_mean/1 -> [CORd_v_CellVoltOfMdl_mean], PowInt/3(CORd_v_CellVoltOfMdl_mean)
  [CORd_v_CellVoltOfMdl_mean] -> EndSoeCalc/3(CORd_v_CellVoltOfMdl_mean)
  CORd_flg_DchEnd/1 -> EndSoeCalc/1(CORd_flg_DchEnd)
  PackDC-IRCalc/2(CORd_r_PackDCIR) -> PowInt/1(CORd_r_PackDCIR)
  CORd_pct_MdlSoc/1 -> PackDC-IRCalc/2(CORd_pct_MdlSoc)
  [CORd_t_MdlTemp] -> EndSoeCalc/4(CORd_t_MdlTemp)
  [IPTd_i_ShuntCur] -> PackDC-IRCalc/3(IPTd_i_ShuntCur)
  PackDC-IRCalc/1(CORd_r_CellDCIR) -> CORd_r_CellDCIR/1
  CORd_t_MdlTemp/1 -> PackDC-IRCalc/1(CORd_t_MdlTemp), [CORd_t_MdlTemp]
  IPTd_i_ShuntCur/1 -> PowInt/4(IPTd_i_ShuntCur), [IPTd_i_ShuntCur]
  PowInt/1(CORd_e_PackSoeRaw1) -> Switch/1
  Divide/1 -> CORd_e_PackSoe/1  "CORd_e_PackSoe"
  [CORd_flg_PackInitStRst] -> Switch1/2
  Switch1/1 -> Divide/1, Unit Delay/1
  [CORd_e_PackSoeInt] -> Switch1/1
  Constant/1 -> Divide/2
  CORd_e_PackSoeInt/1 -> [CORd_e_PackSoeInt]
  CORd_flg_PackInitStRst/1 -> [CORd_flg_PackInitStRst]
  Subtract/1 -> Saturation/1
  Saturation/1 -> Add/2
  Unit Delay/1 -> Subtract/1, Add/1, [CORd_e_PackSoeRawPre]
  Switch/1 -> Subtract/2

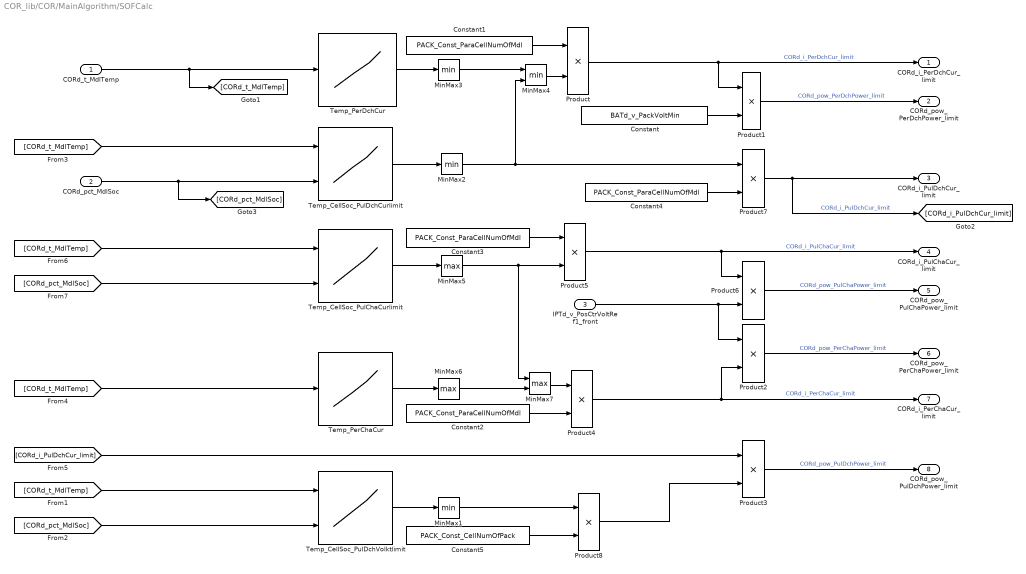
== system COR_lib/COR/MainAlgorithm/SOFCalc ==
  CORd_t_MdlTemp : Inport
  CORd_pct_MdlSoc : Inport  Port=2
  IPTd_v_PosCtrVoltRef1_front : Inport  Port=3
  Constant : Constant  Value=BATd_v_PackVoltMin  OutDataTypeMode=single  OutDataType=fixdt(1, 16)  OutScaling=2^0  OutDataTypeStr=single
  Constant{1..4} (4 alike) : Constant  Value=PACK_Const_ParaCellNumOfMdl  OutDataTypeMode=single  OutDataType=fixdt(1, 16)  OutScaling=2^0  OutDataTypeStr=single
  Constant5 : Constant  Value=PACK_Const_CellNumOfPack  OutDataTypeMode=single  OutDataType=fixdt(1, 16)  OutScaling=2^0  OutDataTypeStr=single
  MinMax1 : MinMax  OutDataType=fixdt(1, 16)  OutScaling=2^0
  MinMax2 : MinMax  OutDataType=fixdt(1, 16)  OutScaling=2^0
  MinMax3 : MinMax  OutDataType=fixdt(1, 16)  OutScaling=2^0
  MinMax4 : MinMax  Inputs=2  OutDataType=fixdt(1, 16)  OutScaling=2^0
  MinMax5 : MinMax  Function=max  OutDataType=fixdt(1, 16)  OutScaling=2^0
  MinMax6 : MinMax  Function=max  OutDataType=fixdt(1, 16)  OutScaling=2^0
  MinMax7 : MinMax  Function=max  Inputs=2  OutDataType=fixdt(1, 16)  OutScaling=2^0
  Product{,1..2,4..7} (7 alike) : Product  OutDataType=fixdt(1, 16)  OutScaling=2^0  RndMeth=Zero
  Product3 : Product  OutDataTypeMode=single  OutDataType=fixdt(1, 16)  OutScaling=2^0  OutDataTypeStr=single  RndMeth=Zero
  Product8 : Product  OutDataTypeMode=single  OutDataType=fixdt(1, 16)  OutScaling=2^0  OutDataTypeStr=single  RndMeth=Zero
  Temp_CellSoc_PulChaCurlimit : Lookup2D  RowIndex=BATx_t_CellDchTemp  ColumnIndex=BATy_pct_CellSoc  Table=BATm_i_PulChaCur_limit
  Temp_CellSoc_PulDchCurlimit : Lookup2D  RowIndex=BATx_t_CellDchTemp  ColumnIndex=BATy_pct_CellSoc  Table=BATm_i_PulDchCur_limit
  Temp_CellSoc_PulDchVolktlimit : Lookup2D  RowIndex=BATx_t_CellDchTemp  ColumnIndex=BATy_pct_CellSoc  Table=BATm_i_PulDchVolt_limit
  Temp_PerChaCur : Lookup  InputValues=BATx_t_CellDchTemp  Table=BATm_i_PerChaCur  LookUpMeth=Interpolation-Use End Values  OutDataType=fixdt(1, 16)  OutScaling=2^0
  Temp_PerDchCur : Lookup  InputValues=BATx_t_CellDchTemp  Table=BATm_i_PerDchCur  LookUpMeth=Interpolation-Use End Values  OutDataType=fixdt(1, 16)  OutScaling=2^0
  CORd_i_PerDchCur_limit : Outport
  CORd_pow_PerDchPower_limit : Outport  Port=2
  CORd_i_PulDchCur_limit : Outport  Port=3
  CORd_i_PulChaCur_limit : Outport  Port=4
  CORd_pow_PulChaPower_limit : Outport  Port=5
  CORd_pow_PerChaPower_limit : Outport  Port=6
  CORd_i_PerChaCur_limit : Outport  Port=7
  CORd_pow_PulDchPower_limit : Outport  Port=8
  wires:
  [CORd_pct_MdlSoc] -> Temp_CellSoc_PulChaCurlimit/2
  [CORd_t_MdlTemp] -> Temp_CellSoc_PulDchCurlimit/1
  [CORd_t_MdlTemp] -> Temp_CellSoc_PulChaCurlimit/1
  MinMax1/1 -> Product8/1
  Product8/1 -> Product3/2
  Constant5/1 -> Product8/2
  Temp_CellSoc_PulDchVolktlimit/1 -> MinMax1/1
  CORd_pct_MdlSoc/1 -> Temp_CellSoc_PulDchCurlimit/2, [CORd_pct_MdlSoc]
  Temp_CellSoc_PulDchCurlimit/1 -> MinMax2/1
  Temp_CellSoc_PulChaCurlimit/1 -> MinMax5/1
  [CORd_t_MdlTemp] -> Temp_CellSoc_PulDchVolktlimit/1
  Temp_PerDchCur/1 -> MinMax3/1
  MinMax2/1 -> MinMax4/2, Product7/1
  MinMax3/1 -> MinMax4/1
  MinMax4/1 -> Product/2
  MinMax5/1 -> MinMax7/1, Product5/2
  [CORd_t_MdlTemp] -> Temp_PerChaCur/1
  Temp_PerChaCur/1 -> MinMax6/1
  MinMax6/1 -> MinMax7/2
  Product1/1 -> CORd_pow_PerDchPower_limit/1  "CORd_pow_PerDchPower_limit"
  Constant/1 -> Product1/2
  Product2/1 -> CORd_pow_PerChaPower_limit/1  "CORd_pow_PerChaPower_limit"
  [CORd_pct_MdlSoc] -> Temp_CellSoc_PulDchVolktlimit/2
  Product3/1 -> CORd_pow_PulDchPower_limit/1  "CORd_pow_PulDchPower_limit"
  Product6/1 -> CORd_pow_PulChaPower_limit/1  "CORd_pow_PulChaPower_limit"
  IPTd_v_PosCtrVoltRef1_front/1 -> Product2/1, Product6/2
  [CORd_i_PulDchCur_limit] -> Product3/1
  Product/1 -> CORd_i_PerDchCur_limit/1, Product1/1  "CORd_i_PerDchCur_limit"
  Constant1/1 -> Product/1
  MinMax7/1 -> Product4/1
  Constant2/1 -> Product4/2
  Product4/1 -> CORd_i_PerChaCur_limit/1, Product2/2  "CORd_i_PerChaCur_limit"
  Constant3/1 -> Product5/1
  Product5/1 -> CORd_i_PulChaCur_limit/1, Product6/1  "CORd_i_PulChaCur_limit"
  Constant4/1 -> Product7/2
  Product7/1 -> [CORd_i_PulDchCur_limit], CORd_i_PulDchCur_limit/1  "CORd_i_PulDchCur_limit"
  CORd_t_MdlTemp/1 -> [CORd_t_MdlTemp], Temp_PerDchCur/1

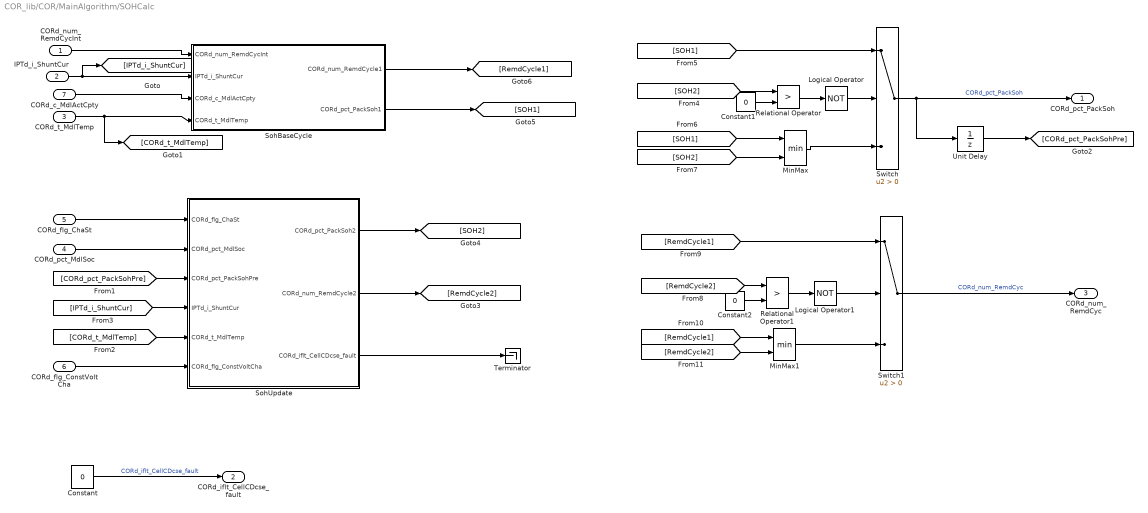
== system COR_lib/COR/MainAlgorithm/SOHCalc ==
  CORd_num_RemdCycInt : Inport
  IPTd_i_ShuntCur : Inport  Port=2
  CORd_t_MdlTemp : Inport  Port=3
  CORd_pct_MdlSoc : Inport  Port=4
  CORd_flg_ChaSt : Inport  Port=5
  CORd_flg_ConstVoltCha : Inport  Port=6
  CORd_c_MdlActCpty : Inport  Port=7
  Constant : Constant  Value=0  OutDataTypeMode=boolean  OutDataType=fixdt(1, 16)  OutScaling=2^0  OutDataTypeStr=boolean
  Constant1 : Constant  Value=0  OutDataTypeMode=boolean  OutDataType=fixdt(1, 16)  OutScaling=2^0  OutDataTypeStr=boolean
  Constant2 : Constant  Value=0  OutDataTypeMode=boolean  OutDataType=fixdt(1, 16)  OutScaling=2^0  OutDataTypeStr=boolean
  Logical Operator : Logic  Operator=NOT  AllPortsSameDT=off  OutDataTypeMode=boolean  LogicDataType=fixdt(0, 8)  OutDataTypeStr=boolean
  Logical Operator1 : Logic  Operator=NOT  AllPortsSameDT=off  OutDataTypeMode=boolean  LogicDataType=fixdt(0, 8)  OutDataTypeStr=boolean
  MinMax : MinMax  Inputs=2  OutDataType=fixdt(1, 16)  OutScaling=2^0
  MinMax1 : MinMax  Inputs=2  OutDataType=fixdt(1, 16)  OutScaling=2^0
  Relational Operator : RelationalOperator  Operator=>  LogicOutDataTypeMode=boolean  LogicDataType=fixdt(0, 8)  OutDataTypeStr=boolean
  Relational Operator1 : RelationalOperator  Operator=>  LogicOutDataTypeMode=boolean  LogicDataType=fixdt(0, 8)  OutDataTypeStr=boolean
  SohBaseCycle : Subsystem
  SohUpdate : Subsystem
  Switch : Switch  Criteria=u2 > Threshold  OutDataType=fixdt(1, 16)  OutScaling=2^0
  Switch1 : Switch  Criteria=u2 > Threshold  OutDataType=fixdt(1, 16)  OutScaling=2^0
  Terminator : Terminator
  Unit Delay : UnitDelay  SampleTime=-1
  CORd_pct_PackSoh : Outport
  CORd_iflt_CellCDcse_fault : Outport  Port=2  OutDataType=fixdt(1, 16)  OutScaling=2^0
  CORd_num_RemdCyc : Outport  Port=3
  wires:
  IPTd_i_ShuntCur/1 -> [IPTd_i_ShuntCur], SohBaseCycle/2(IPTd_i_ShuntCur)
  Logical Operator/1 -> Switch/2
  Switch/1 -> Unit Delay/1, CORd_pct_PackSoh/1  "CORd_pct_PackSoh"
  Constant1/1 -> Relational Operator/2
  Relational Operator/1 -> Logical Operator/1
  [SOH2] -> Relational Operator/1
  Constant/1 -> CORd_iflt_CellCDcse_fault/1  "CORd_iflt_CellCDcse_fault"
  SohUpdate/3(CORd_iflt_CellCDcse_fault) -> Terminator/1
  CORd_flg_ConstVoltCha/1 -> SohUpdate/6(CORd_flg_ConstVoltCha)
  [CORd_t_MdlTemp] -> SohUpdate/5(CORd_t_MdlTemp)
  [IPTd_i_ShuntCur] -> SohUpdate/4(IPTd_i_ShuntCur)
  [CORd_pct_PackSohPre] -> SohUpdate/3(CORd_pct_PackSohPre)
  CORd_pct_MdlSoc/1 -> SohUpdate/2(CORd_pct_MdlSoc)
  CORd_flg_ChaSt/1 -> SohUpdate/1(CORd_flg_ChaSt)
  Unit Delay/1 -> [CORd_pct_PackSohPre]
  SohUpdate/1(CORd_pct_PackSoh2) -> [SOH2]
  CORd_num_RemdCycInt/1 -> SohBaseCycle/1(CORd_num_RemdCycInt)
  CORd_t_MdlTemp/1 -> [CORd_t_MdlTemp], SohBaseCycle/4(CORd_t_MdlTemp)
  CORd_c_MdlActCpty/1 -> SohBaseCycle/3(CORd_c_MdlActCpty)
  SohUpdate/2(CORd_num_RemdCycle2) -> [RemdCycle2]
  SohBaseCycle/2(CORd_pct_PackSoh1) -> [SOH1]
  SohBaseCycle/1(CORd_num_RemdCycle1) -> [RemdCycle1]
  [SOH1] -> Switch/1
  [SOH1] -> MinMax/1
  [SOH2] -> MinMax/2
  MinMax/1 -> Switch/3
  Logical Operator1/1 -> Switch1/2
  Switch1/1 -> CORd_num_RemdCyc/1  "CORd_num_RemdCyc"
  Constant2/1 -> Relational Operator1/2
  Relational Operator1/1 -> Logical Operator1/1
  [RemdCycle2] -> Relational Operator1/1
  [RemdCycle1] -> Switch1/1
  [RemdCycle1] -> MinMax1/1
  [RemdCycle2] -> MinMax1/2
  MinMax1/1 -> Switch1/3

== system COR_lib/COR/MainAlgorithm/Timer ==
  Add : Sum  OutDataType=fixdt(1, 16)  OutScaling=2^-10
  Constant : Constant  OutDataType=fixdt(1, 16)  OutScaling=2^0
  Constant1 : Constant  Value=30  OutDataType=fixdt(1, 16)  OutScaling=2^0
  Constant2 : Constant  Value=0  OutDataType=fixdt(1, 16)  OutScaling=2^0
  Constant3 : Constant  Value=29  OutDataType=fixdt(1, 16)  OutScaling=2^0
  Relational Operator : RelationalOperator  Operator===  LogicOutDataTypeMode=boolean  LogicDataType=fixdt(0, 8)  OutDataTypeStr=boolean
  Relational Operator2 : RelationalOperator  Operator=~=  LogicOutDataTypeMode=boolean  LogicDataType=fixdt(0, 8)  OutDataTypeStr=boolean
  Switch : Switch  Criteria=u2 > Threshold  OutDataType=fixdt(1, 16)  OutScaling=2^0
  Unit Delay1 : UnitDelay  SampleTime=-1
  Cord_enum_Timer_300ms : Outport  OutDataType=fixdt(1, 16)  OutScaling=2^0
  wires:
  Constant/1 -> Add/2
  Add/1 -> Relational Operator2/1, Switch/1
  Constant1/1 -> Relational Operator2/2
  Relational Operator2/1 -> Switch/2
  Constant2/1 -> Switch/3
  Switch/1 -> Unit Delay1/1, Relational Operator/1
  Unit Delay1/1 -> Add/1
  Relational Operator/1 -> Cord_enum_Timer_300ms/1
  Constant3/1 -> Relational Operator/2

== system COR_lib/COR/MainAlgorithm/CellOhmRObs/CellOhmRCal ==
  IPTd_i_ShuntCur : Inport
  CORd_v_CellVoltOfMdl_mean : Inport  Port=2
  CORd_pct_CellSoc : Inport  Port=3
  CORd_t_CellTemp : Inport  Port=4
  Abs : Abs  OutDataType=fixdt(1, 16)  OutScaling=2^0
  Abs1 : Abs  OutDataType=fixdt(1, 16)  OutScaling=2^0
  Add : Sum  Inputs=+-  OutDataType=fixdt(1, 16)  OutScaling=2^-10
  Constant1 : Constant  Value=10  OutDataType=fixdt(1, 16)  OutScaling=2^0
  Relational Operator : RelationalOperator  LogicOutDataTypeMode=boolean  LogicDataType=fixdt(0, 8)  OutDataTypeStr=boolean
  Subsystem : Subsystem
  Unit Delay : UnitDelay  SampleTime=-1
  CORd_r_CellOhmR : Outport  OutDataType=fixdt(1, 16)  OutScaling=2^0
  wires:
  Subsystem/1(CORd_r_CellOhmR) -> CORd_r_CellOhmR/1
  CORd_v_CellVoltOfMdl_mean/1 -> Subsystem/2(CORd_v_CellVoltOfMdl_Mean)
  CORd_t_CellTemp/1 -> Subsystem/3(CORd_t_CellTemp)
  CORd_pct_CellSoc/1 -> Subsystem/4(CORd_pct_CellSoc)
  IPTd_i_ShuntCur/1 -> Abs1/1
  Unit Delay/1 -> Add/2
  Constant1/1 -> Relational Operator/2
  Relational Operator/1 -> Subsystem/Enable
  Abs/1 -> Relational Operator/1
  Abs1/1 -> Add/1, Unit Delay/1
  Add/1 -> Abs/1, Subsystem/1(CORd_i_CurSnrDelta)

== system COR_lib/COR/MainAlgorithm/CellOhmRObs/CellOhmRObs ==
  CORd_r_CellOhmR : Inport
  CORd_r_CellOhmRInt : Inport  Port=2
  Enable : EnablePort
  Constant1 : Constant  Value=CORc_fac_CellRDcse_fault  OutDataTypeMode=single  OutDataType=fixdt(1, 16)  OutScaling=2^0  OutDataTypeStr=single
  Constant8 : Constant  Value=CORc_fac_CellRDcse_warn  OutDataTypeMode=single  OutDataType=fixdt(1, 16)  OutScaling=2^0  OutDataTypeStr=single
  MinMax : MinMax  OutDataType=fixdt(1, 16)  OutScaling=2^0
  MinMax1 : MinMax  Function=max  OutDataType=fixdt(1, 16)  OutScaling=2^0
  MinMax2 : MinMax  OutDataType=fixdt(1, 16)  OutScaling=2^0
  MinMax3 : MinMax  Function=max  OutDataType=fixdt(1, 16)  OutScaling=2^0
  Product1 : Product  OutDataType=fixdt(1, 16)  OutScaling=2^0  RndMeth=Zero
  Product2 : Product  OutDataType=fixdt(1, 16)  OutScaling=2^0  RndMeth=Zero
  Relational Operator1 : RelationalOperator  Operator=>  LogicOutDataTypeMode=boolean  LogicDataType=fixdt(0, 8)  OutDataTypeStr=boolean
  Relational Operator2 : RelationalOperator  Operator=<  LogicOutDataTypeMode=boolean  LogicDataType=fixdt(0, 8)  OutDataTypeStr=boolean
  CORd_iflt_CellRDcse_fault : Outport  OutDataType=fixdt(1, 16)  OutScaling=2^0
  CORd_iflt_CellRIcse_fault : Outport  Port=2  OutDataType=fixdt(1, 16)  OutScaling=2^0
  wires:
  Relational Operator2/1 -> CORd_iflt_CellRDcse_fault/1
  Relational Operator1/1 -> CORd_iflt_CellRIcse_fault/1
  Constant8/1 -> Product2/2
  [CORd_r_CellOhmR] -> MinMax1/1
  Product2/1 -> MinMax3/1
  Product1/1 -> MinMax2/1
  MinMax/1 -> Relational Operator2/1
  MinMax1/1 -> Relational Operator1/1
  CORd_r_CellOhmR/1 -> MinMax/1, [CORd_r_CellOhmR]
  Constant1/1 -> Product1/1
  CORd_r_CellOhmRInt/1 -> Product2/1, Product1/2
  MinMax2/1 -> Relational Operator2/2
  MinMax3/1 -> Relational Operator1/2

== system COR_lib/COR/MainAlgorithm/CellOhmRObs/Timer ==
  Constant : Constant  OutDataType=fixdt(1, 16)  OutScaling=2^0
  Constant1 : Constant  Value=40  OutDataType=fixdt(1, 16)  OutScaling=2^0
  Relational Operator : RelationalOperator  Operator=>  LogicOutDataTypeMode=boolean  LogicDataType=fixdt(0, 8)  OutDataTypeStr=boolean
  integrator : Defined_Functionality/integrator  SystemSampleTime=-1  Initial_Value=0
  Cord_flag_CellOhmRObs : Outport  OutDataType=fixdt(1, 16)  OutScaling=2^0
  wires:
  Constant/1 -> integrator/1
  integrator/1 -> Relational Operator/1
  Relational Operator/1 -> Cord_flag_CellOhmRObs/1
  Constant1/1 -> Relational Operator/2

== system COR_lib/COR/MainAlgorithm/SOCCalc/ChaEnd ==
  IPTd_i_ShuntCur : Inport
  CORd_pct_MdlSocPre : Inport  Port=2
  Abs : Abs  OutDataType=fixdt(1, 16)  OutScaling=2^0
  Constant : Constant  Value=CORc_i_SOCCrectCurThrld  OutDataTypeMode=single  OutDataType=fixdt(1, 16)  OutScaling=2^0  OutDataTypeStr=single
  Constant1 : Constant  Value=0.3  OutDataType=fixdt(1, 16)  OutScaling=2^0
  Constant2 : Constant  Value=0  OutDataType=fixdt(1, 16)  OutScaling=2^0
  Constant3 : Constant  Value=0.8  OutDataType=fixdt(1, 16)  OutScaling=2^0
  Constant4 : Constant  Value=0  OutDataType=fixdt(1, 16)  OutScaling=2^0
  Logical Operator : Logic  AllPortsSameDT=off  OutDataTypeMode=boolean  LogicDataType=fixdt(0, 8)  OutDataTypeStr=boolean
  Logical Operator1 : Logic  AllPortsSameDT=off  OutDataTypeMode=boolean  LogicDataType=fixdt(0, 8)  OutDataTypeStr=boolean
  Logical Operator2 : Logic  Operator=OR  AllPortsSameDT=off  OutDataTypeMode=boolean  LogicDataType=fixdt(0, 8)  OutDataTypeStr=boolean
  Logical Operator3 : Logic  AllPortsSameDT=off  OutDataTypeMode=boolean  LogicDataType=fixdt(0, 8)  OutDataTypeStr=boolean
  MinMax1 : MinMax  OutDataType=fixdt(1, 16)  OutScaling=2^0
  Relational Operator : RelationalOperator  Operator=<=  LogicOutDataTypeMode=boolean  LogicDataType=fixdt(0, 8)  OutDataTypeStr=boolean
  Relational Operator1 : RelationalOperator  Operator=>  LogicOutDataTypeMode=boolean  LogicDataType=fixdt(0, 8)  OutDataTypeStr=boolean
  Relational Operator2 : RelationalOperator  LogicOutDataTypeMode=boolean  LogicDataType=fixdt(0, 8)  OutDataTypeStr=boolean
  Relational Operator3 : RelationalOperator  Operator=<  LogicOutDataTypeMode=boolean  LogicDataType=fixdt(0, 8)  OutDataTypeStr=boolean
  Relational Operator4 : RelationalOperator  Operator=<=  LogicOutDataTypeMode=boolean  LogicDataType=fixdt(0, 8)  OutDataTypeStr=boolean
  Subtract : Sum  Inputs=+-  OutDataType=fixdt(1, 16)  OutScaling=2^-10
  average : Defined_Functionality/average  SystemSampleTime=-1  time=2000  period=10
      settings: AttributesFormatString=[TIME_ms=%<time>]\n[PERIOD_ms=%<period>]
  CORd_flg_DchEnd : Outport
  CORd_flg_SOCCrect : Outport  Port=2
  CORd_i_ShuntCur_mean : Outport  Port=3
  wires:
  MinMax1/1 -> Relational Operator2/1, Relational Operator/1
  [IPTd_i_ShuntCur] -> average/1, Subtract/1, Relational Operator3/1
  average/1 -> CORd_i_ShuntCur_mean/1, Subtract/2  "CORd_i_ShuntCur_mean"
  Logical Operator3/1 -> CORd_flg_SOCCrect/1  "CORd_flg_SOCCrect"
  Relational Operator4/1 -> Logical Operator3/2
  Constant/1 -> Relational Operator4/2
  Abs/1 -> Relational Operator4/1
  Subtract/1 -> Abs/1
  Logical Operator2/1 -> Logical Operator3/1
  Constant1/1 -> Relational Operator/2
  Constant2/1 -> Relational Operator1/2
  CORd_pct_MdlSocPre/1 -> MinMax1/1
  Logical Operator/1 -> CORd_flg_DchEnd/1, Logical Operator2/1  "CORd_flg_DchEnd"
  IPTd_i_ShuntCur/1 -> [IPTd_i_ShuntCur], Relational Operator1/1
  Constant3/1 -> Relational Operator2/2
  Relational Operator2/1 -> Logical Operator1/1
  Constant4/1 -> Relational Operator3/2
  Relational Operator3/1 -> Logical Operator1/2
  Logical Operator1/1 -> Logical Operator2/2
  Relational Operator1/1 -> Logical Operator/1
  Relational Operator/1 -> Logical Operator/2
